simulink model "KITTDynamicsFinal"  (R2014b)
settings: Solver=ode45  StartTime=0.0  StopTime=8.0  MaxStep=0.01  RelTol=1e-3
values from neighbouring files (symbols this model uses):
  D_intersect = polyxpoly(T1,Y1,T2,Y2)    [KITTDriver.m]
  V_ini = V_ini  + 0.1    (= 16.6666666667)    [KITTDriver.m]
undefined symbols (not defined in the file or in its folder): b, c, Fa_max, Fb_max, m
libraries: simulink x2
settings Model: Creator=Martijn  LastModifiedBy=Martijn
settings DataIOCC: LimitDataPoints=off

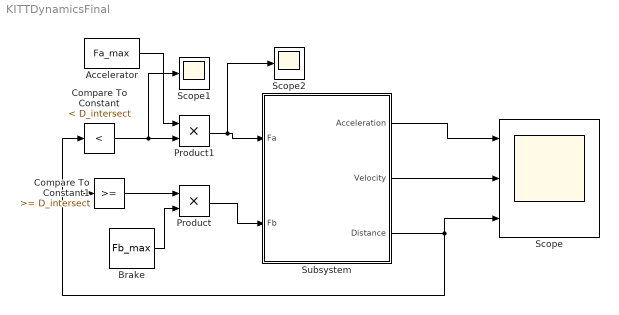
== system KITTDynamicsFinal ==
  Accelerator : Constant  Value=Fa_max
  Brake : Constant  Value=Fb_max
  Compare To Constant : simulink/Logic and Bit Operations/Compare To Constant  relop=<  const=D_intersect  OutDataTypeStr=boolean
  Compare To Constant1 : simulink/Logic and Bit Operations/Compare To Constant  relop=>=  const=D_intersect  OutDataTypeStr=boolean
  Product : Product
  Product1 : Product
  Scope : Scope  NumInputPorts=3
      settings: YMin=-10~-5~-5  YMax=10~5~5
  Scope1 : Scope
  Scope2 : Scope
      settings: SaveName=ScopeData2
  Subsystem : Subsystem
  wires:
  Subsystem/1(Acceleration) -> Scope/1
  Subsystem/2(Velocity) -> Scope/2
  Brake/1 -> Product/2
  Product/1 -> Subsystem/2(Fb)
  Subsystem/3("Distance ") -> Compare To Constant1/1, Compare To Constant/1, Scope/3
  Accelerator/1 -> Product1/1
  Product1/1 -> Scope2/1, Subsystem/1(Fa)
  Compare To Constant/1 -> Product1/2, Scope1/1
  Compare To Constant1/1 -> Product/1

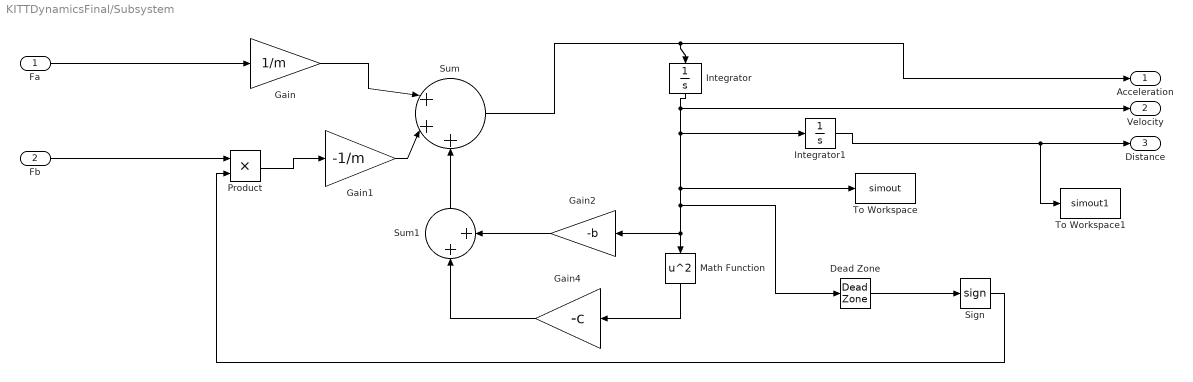
== system KITTDynamicsFinal/Subsystem ==
  Fa : Inport
  Fb : Inport  Port=2
  Dead Zone : DeadZone  LowerValue=-0.001  UpperValue=0.001  SaturateOnIntegerOverflow=on
  Gain : Gain  Gain=1/m
  Gain1 : Gain  Gain=-1/m
  Gain2 : Gain  Gain=-b
  Gain4 : Gain  Gain=-c
  Integrator : Integrator  InitialCondition=V_ini
  Integrator1 : Integrator
  Math Function : Math  Operator=square  SaturateOnIntegerOverflow=on
  Product : Product
  Sign : Signum
  Sum : Sum  Inputs=|+++
  Sum1 : Sum  Inputs=|++
  To Workspace : ToWorkspace  VariableName=simout  SaveFormat=Structure With Time  SampleTime=-1
  To Workspace1 : ToWorkspace  VariableName=simout1  SaveFormat=Structure With Time  SampleTime=-1
  Acceleration : Outport
  Velocity : Outport  Port=2
  "Distance " : Outport  Port=3
  wires:
  Gain1/1 -> Sum/2
  Gain/1 -> Sum/1
  Gain2/1 -> Sum1/2
  Sum1/1 -> Sum/3
  Integrator/1 -> Integrator1/1, To Workspace/1, Dead Zone/1, Math Function/1, Gain2/1, Velocity/1
  Math Function/1 -> Gain4/1
  Sign/1 -> Product/2
  Integrator1/1 -> To Workspace1/1, "Distance "/1
  Gain4/1 -> Sum1/1
  Sum/1 -> Acceleration/1, Integrator/1
  Fa/1 -> Gain/1
  Fb/1 -> Product/1
  Product/1 -> Gain1/1
  Dead Zone/1 -> Sign/1
